simulink subsystem "subsystem_staticFriction"  (R2022a)
settings: Solver=VariableStepAuto  StartTime=0.0  StopTime=10.0  RelTol=1e-3
settings Model: Creator=Philipp  LastModifiedBy=Philipp
settings DebuggingCC: UnconnectedInputMsg=warning  UnconnectedOutputMsg=warning  UnconnectedLineMsg=warning
settings RTWCC: DLArmComputeVersion=19.05

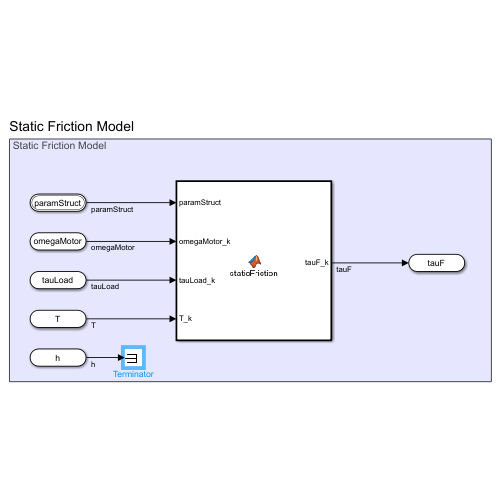
[thumbnail: Simulink's stored preview of the top-level diagram]
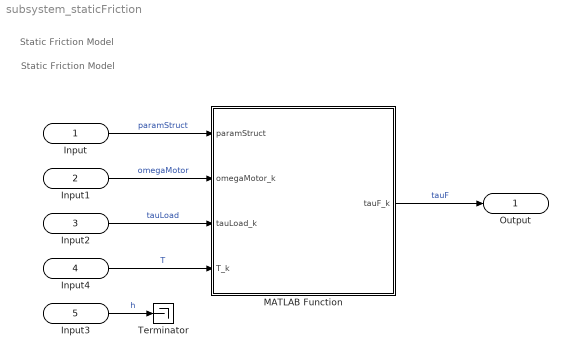
== system subsystem_staticFriction ==
  note: Static Friction Model
  note: Static Friction Model
  Input : Inport  OutDataTypeStr=Bus: main_bus
  Input1 : Inport  Port=2
  Input2 : Inport  Port=3  PortDimensions=3
  Input4 : Inport  Port=4
  Input3 : Inport  Port=5
  MATLAB Function : MATLAB Function  TreatAsAtomicUnit=on
  Terminator : Terminator
  Output : Outport
  wires:
  Input3/1 -> Terminator/1  "h"
  MATLAB Function/1(tauF_k) -> Output/1  "tauF"
  Input2/1 -> MATLAB Function/3(tauLoad_k)  "tauLoad"
  Input4/1 -> MATLAB Function/4(T_k)  "T"
  Input/1 -> MATLAB Function/1(paramStruct)  "paramStruct"
  Input1/1 -> MATLAB Function/2(omegaMotor_k)  "omegaMotor"

== matlab function subsystem_staticFriction/MATLAB Function ==
  data: paramStruct input; omegaMotor_k input; tauLoad_k input; tauF_k output; T_k input
function tauF_k= staticFriction(paramStruct, omegaMotor_k, tauLoad_k, T_k)

i_g = paramStruct.robot.i_g;

% Convert to deg
omegaMotorDeg_k = omegaMotor_k .* (180/pi);

tauF_k = staticFriction_model(paramStruct, omegaMotorDeg_k, tauLoad_k./i_g, T_k);
tauF_k = tauF_k .* i_g;
